simulink model "schema_di_controlloC1_Pelliccia_Tornabene_Valmaggi_PtiOpz"  (R2023b)
settings: Solver=VariableStepAuto  StartTime=0.0  StopTime=0.2  RelTol=1e-3
values from neighbouring files (symbols this model uses):
  C = [1 0]    [CAT_ProgettoC1_Tornabene_Valmaggi_Pelliccia.m]
  DD = 1    [CAT_ProgettoC1_Tornabene_Valmaggi_Pelliccia.m]
  kk = 1:4    [CAT_ProgettoC1_Tornabene_Valmaggi_Pelliccia.m]
  NN = 0.2    [CAT_ProgettoC1_Tornabene_Valmaggi_Pelliccia.m]
  omega_d = 0.01    [CAT_ProgettoC1_Tornabene_Valmaggi_Pelliccia.m]
  omega_n = omega_n_min    (= 80000)    [CAT_ProgettoC1_Tornabene_Valmaggi_Pelliccia.m]
  u_e = m*9.81 + k*x1_e    (= 199525)    [CAT_ProgettoC1_Tornabene_Valmaggi_Pelliccia.m]
  WW = 1    [CAT_ProgettoC1_Tornabene_Valmaggi_Pelliccia.m]
  x1_e = 0.35    [CAT_ProgettoC1_Tornabene_Valmaggi_Pelliccia.m]
  x1_value = x1_e    (= 0.35)    [CAT_ProgettoC1_Tornabene_Valmaggi_Pelliccia.m]
  x2_value = x2_e    (= 0)    [CAT_ProgettoC1_Tornabene_Valmaggi_Pelliccia.m]
libraries: cstblocks x1
settings Model: Creator=enrico  LastModifiedBy=enrico

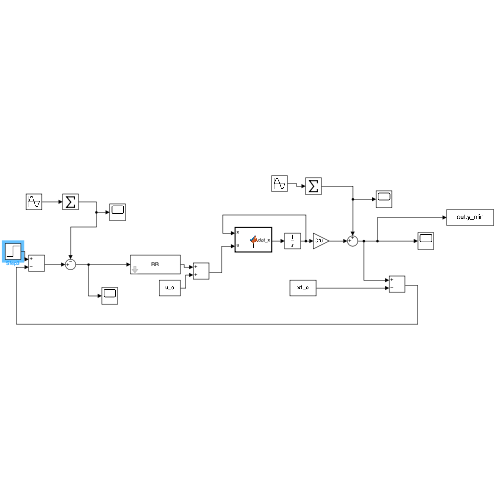
[thumbnail: Simulink's stored preview of the top-level diagram]
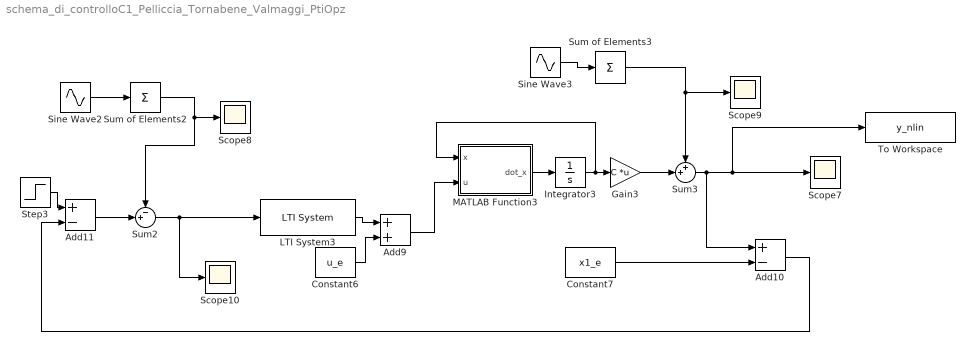
== system schema_di_controlloC1_Pelliccia_Tornabene_Valmaggi_PtiOpz ==
  Add10 : Sum  Inputs=+-
  Add11 : Sum  Inputs=+-
  Add9 : Sum
  Constant6 : Constant  Value=u_e
  Constant7 : Constant  Value=x1_e
  Gain3 : Gain  Gain=C  Multiplication=Matrix(K*u)
  Integrator3 : Integrator  InitialCondition=[x1_value; x2_value]
  LTI System3 : cstblocks/LTI System  sys=RR  IC=[]  PadeOrder=0
  MATLAB Function3 : MATLAB Function  TreatAsAtomicUnit=on
  Scope{7..10} (4 alike) : Scope
  Sine Wave2 : Sin  Amplitude=NN  Frequency=omega_n*kk  SampleTime=0
  Sine Wave3 : Sin  Amplitude=DD  Frequency=omega_d*kk  SampleTime=0
  Step3 : Step  Time=0  After=WW  SampleTime=0
  Sum of Elements2 : Sum  Inputs=+
  Sum of Elements3 : Sum  Inputs=+  CollapseDim=4
  Sum2 : Sum  Inputs=-+|
  Sum3 : Sum  Inputs=++|
  To Workspace : ToWorkspace  VariableName=y_nlin  SaveFormat=Timeseries  SampleTime=-1
  wires:
  Integrator3/1 -> MATLAB Function3/1(x), Gain3/1
  LTI System3/1 -> Add9/1
  MATLAB Function3/1(dot_x) -> Integrator3/1
  Add10/1 -> Add11/2
  Sum2/1 -> Scope10/1, LTI System3/1
  Constant6/1 -> Add9/2
  Sum of Elements2/1 -> Sum2/1, Scope8/1
  Add11/1 -> Sum2/2
  Add9/1 -> MATLAB Function3/2(u)
  Constant7/1 -> Add10/2
  Step3/1 -> Add11/1
  Sum3/1 -> To Workspace/1, Scope7/1, Add10/1
  Sine Wave2/1 -> Sum of Elements2/1
  Sum of Elements3/1 -> Scope9/1, Sum3/1
  Gain3/1 -> Sum3/2
  Sine Wave3/1 -> Sum of Elements3/1

== matlab function schema_di_controlloC1_Pelliccia_Tornabene_Valmaggi_PtiOpz/MATLAB Function3 ==
  data: x input; u input; dot_x output
function dot_x = f(x,u)

m = 2500;   % Massa
beta = 0.1; % Coefficiente di non linearità della molla
n = 3;      % Coefficiente di non linearità della molla
k = 5 * 1e5;% Costante elastica lineare della molla
b = 350;    % Coefficiente di attrito dinamico
g = 9.81;   % Acc. gravitazionale

dot_x = zeros(2,1);
dot_x(1) = x(2);
dot_x(2) = - g - (b/m) * x(2) - (k/m) * x(1) - (beta/m) * (x(2)^3 + n * x(2) * sin(n*x(2))^2 ) + (u / m);
